simulink model "capitol8prob2"  (R2013a)
settings: Solver=ode45  StartTime=0.0  StopTime=1000  RelTol=1e-3
undefined symbols (not defined in the file): des, gcbh
settings Model: Creator=user  LastModifiedBy=user

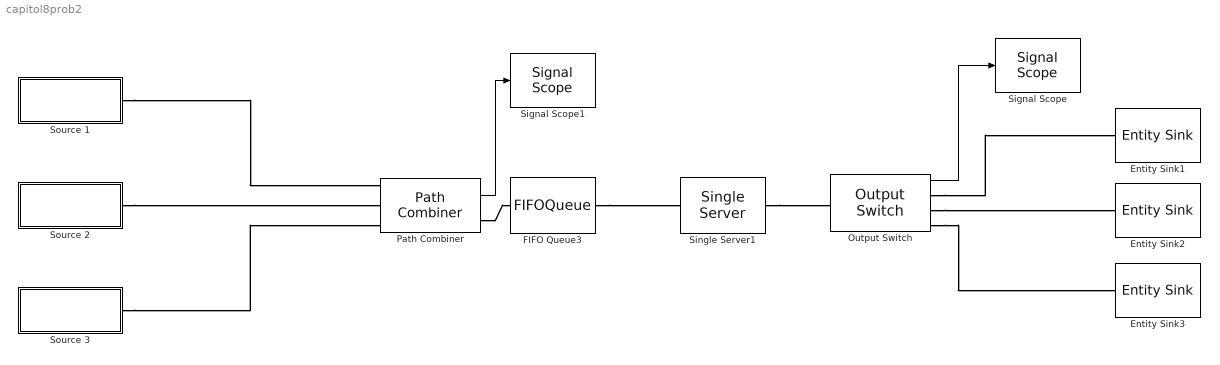
== system capitol8prob2 ==
  Entity Sink1 : EntitySink
  Entity Sink2 : EntitySink
  Entity Sink3 : EntitySink
  FIFO Queue3 : FIFOQueue
  Output Switch : OutputSwitch  SwitchingCriterion=From attribute  AttributeName=Destination  StatLastDeparturePort=on
      settings: OutputPortMap=o3
  Path Combiner : PathCombiner  InputPortPrecedence=Round robin  StatLastArrivalPort=on
      settings: OutputPortMap=o1
  Signal Scope : SignalScope  LoadFcn=des.scope.CallbackSupport('seLoadFcn',gcbh)  StartFcn=des.scope.CallbackSupport('seStartFcn',gcbh)  StopFcn=des.scope.CallbackSupport('seStopFcn',gcbh)
      settings: CopyFcn=des.scope.CallbackSupport('seCopyFcn',gcbh)  DeleteFcn=des.scope.CallbackSupport('seDeleteFcn',gcbh)  PreSaveFcn=des.scope.CallbackSupport('sePreSaveFcn',gcbh)  NameChangeFcn=des.scope.CallbackSupport('seNameChangeFcn',gcbh)  OpenFcn=des.scope.CallbackSupport('seOpenFcn',gcbh)
  Signal Scope1 : SignalScope  LoadFcn=des.scope.CallbackSupport('seLoadFcn',gcbh)  StartFcn=des.scope.CallbackSupport('seStartFcn',gcbh)  StopFcn=des.scope.CallbackSupport('seStopFcn',gcbh)
      settings: CopyFcn=des.scope.CallbackSupport('seCopyFcn',gcbh)  DeleteFcn=des.scope.CallbackSupport('seDeleteFcn',gcbh)  PreSaveFcn=des.scope.CallbackSupport('sePreSaveFcn',gcbh)  NameChangeFcn=des.scope.CallbackSupport('seNameChangeFcn',gcbh)  OpenFcn=des.scope.CallbackSupport('seOpenFcn',gcbh)
  Single Server1 : SingleServer
  Source 1 : Subsystem
  Source 2 : Subsystem
  Source 3 : Subsystem
  wires:
  Path Combiner/1 -> Signal Scope1/1
  Output Switch/1 -> Signal Scope/1
  connections:
  Single Server1/RConn1 -- Output Switch/LConn1
  Source 3/LConn1 -- Path Combiner/LConn3
  Output Switch/RConn1 -- Entity Sink1/LConn1
  Output Switch/RConn2 -- Entity Sink2/LConn1
  Source 2/RConn1 -- Path Combiner/LConn2
  Path Combiner/RConn1 -- FIFO Queue3/LConn1
  Source 1/LConn1 -- Path Combiner/LConn1
  FIFO Queue3/RConn1 -- Single Server1/LConn1
  Output Switch/RConn3 -- Entity Sink3/LConn1

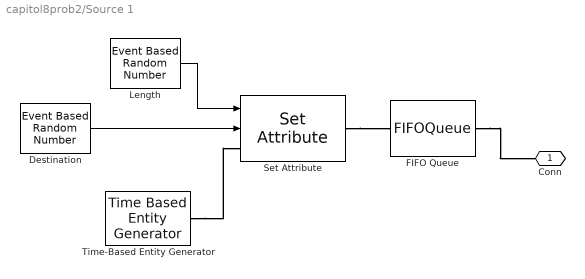
== system capitol8prob2/Source 1 ==
  Destination : EventBasedRandomNumber  Distribution=Discrete uniform  minUnid=1  maxUnid=3  numValueUnid=3
  FIFO Queue : FIFOQueue
  Length : EventBasedRandomNumber  Distribution=Discrete uniform  minUnif=6  maxUnif=10  minUnid=6  maxUnid=10  numValueUnid=5  Seed=4324234
  Set Attribute : SetAttribute  AttributeName=Lenght|Destination  AttributeFrom=Signal port|Signal port  AttributeValue=1|1  AttributeTreatAsVector=1|1  EvaluatedAttributeValue={ [];[]}
      settings: InputPortMap=u0,u1
  Time-Based Entity Generator : TimeBasedEntityGenerator
  Conn : PMIOPort  Port=1  Side=Left
  wires:
  Destination/1 -> Set Attribute/2
  Length/1 -> Set Attribute/1
  connections:
  Time-Based Entity Generator/RConn1 -- Set Attribute/LConn1
  Set Attribute/RConn1 -- FIFO Queue/LConn1
  FIFO Queue/RConn1 -- Conn/RConn1

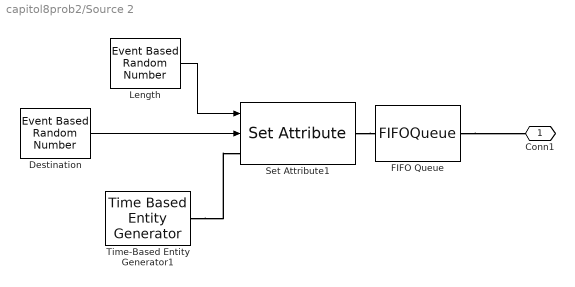
== system capitol8prob2/Source 2 ==
  Destination : EventBasedRandomNumber  Distribution=Discrete uniform  minUnid=1  maxUnid=3  numValueUnid=3
  FIFO Queue : FIFOQueue
  Length : EventBasedRandomNumber  Distribution=Discrete uniform  minUnif=6  maxUnif=10  minUnid=6  maxUnid=10  numValueUnid=5  Seed=4324234
  Set Attribute1 : SetAttribute  AttributeName=Lenght|Destination  AttributeFrom=Signal port|Signal port  AttributeValue=1|1  AttributeTreatAsVector=1|1  EvaluatedAttributeValue={ [];[]}
      settings: InputPortMap=u0,u1
  Time-Based Entity Generator1 : TimeBasedEntityGenerator
  Conn1 : PMIOPort  Port=1  Side=Right
  wires:
  Destination/1 -> Set Attribute1/2
  Length/1 -> Set Attribute1/1
  connections:
  Time-Based Entity Generator1/RConn1 -- Set Attribute1/LConn1
  FIFO Queue/RConn1 -- Conn1/RConn1
  Set Attribute1/RConn1 -- FIFO Queue/LConn1

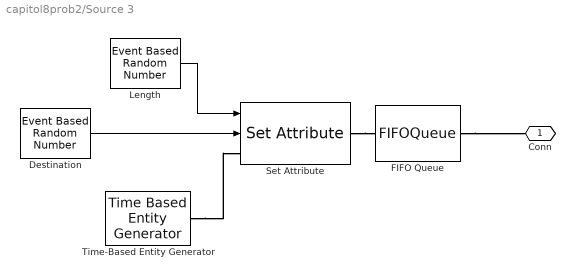
== system capitol8prob2/Source 3 ==
  Destination : EventBasedRandomNumber  Distribution=Discrete uniform  minUnid=1  maxUnid=3  numValueUnid=3
  FIFO Queue : FIFOQueue
  Length : EventBasedRandomNumber  Distribution=Discrete uniform  minUnif=6  maxUnif=10  minUnid=6  maxUnid=10  numValueUnid=5  Seed=4324234
  Set Attribute : SetAttribute  AttributeName=Lenght|Destination  AttributeFrom=Signal port|Signal port  AttributeValue=1|1  AttributeTreatAsVector=1|1  EvaluatedAttributeValue={ [];[]}
      settings: InputPortMap=u0,u1
  Time-Based Entity Generator : TimeBasedEntityGenerator
  Conn : PMIOPort  Port=1  Side=Left
  wires:
  Destination/1 -> Set Attribute/2
  Length/1 -> Set Attribute/1
  connections:
  Time-Based Entity Generator/RConn1 -- Set Attribute/LConn1
  FIFO Queue/RConn1 -- Conn/RConn1
  Set Attribute/RConn1 -- FIFO Queue/LConn1
